simulink model "PrinterRC_SIM"  (Simulink 7.8)
settings: Solver=FixedStepDiscrete  StartTime=0.0  StopTime=30  FixedStep=1/1000  RelTol=1e-3
InitFcn:
  | load('Exp_RC_settings.mat');
values from neighbouring files (symbols this model uses):
  N = length(r)    [SimExpRC_SPERTE.m]
  N_RC_activate = 5    [SimExpRC_SPERTE.m]
  N_trial = 50    [SimExpRC_SPERTE.m]
  p_Q = M    (= 50)    [DesignControllerRC.m]
undefined symbols (not defined in the file or in its folder): p_L, r
libraries: simulink x4, cstblocks x3
settings Model: Creator=jbolder  LastModifiedBy=lblanken
settings DebuggingCC: FrameProcessingCompatibilityMsg=error
settings CodeAppCC: CustomSymbolStrType=$N$R$M_T
settings GRTTargetCC: TargetFunctionLibrary=C89/C90 (ANSI)

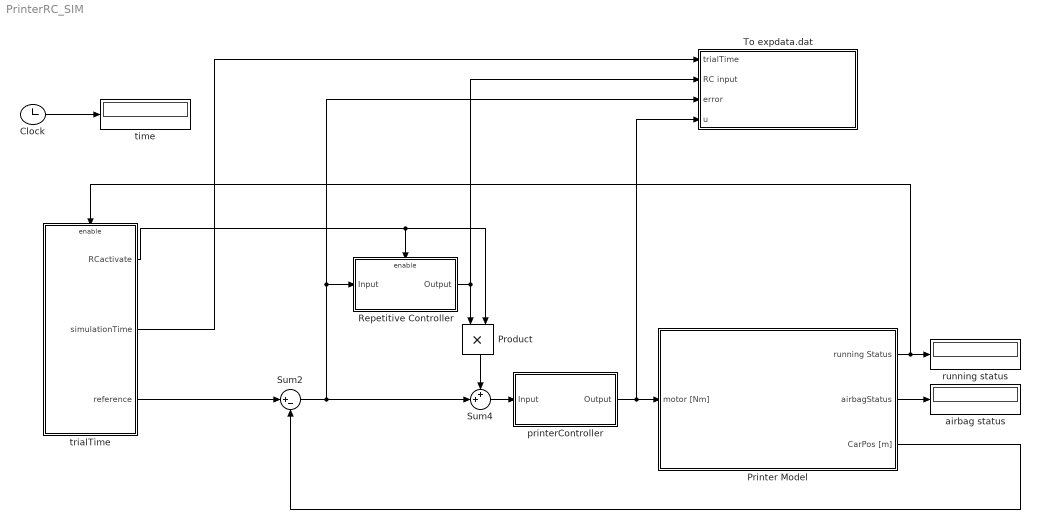
== system PrinterRC_SIM ==
  Clock : Clock
  Printer Model : Subsystem  InitFcn=load('PrinterModel.mat');
  Product : Product
  Repetitive Controller : Subsystem  InitFcn=load('RCController.mat');
  Sum2 : Sum  Inputs=|+-
  Sum4 : Sum  Inputs=++|  SaturateOnIntegerOverflow=on  InputSameDT=on  OutDataTypeStr=Inherit: Same as first input
  To expdata.dat : Subsystem
  airbag status : Display
      settings: Decimation=50
  printerController : Subsystem
  running status : Display
      settings: Decimation=50
  time : Display
      settings: Decimation=50
  trialTime : Subsystem  TreatAsAtomicUnit=on
  wires:
  trialTime/3(reference) -> Sum2/1
  Clock/1 -> time/1
  Printer Model/3(CarPos [m]) -> Sum2/2
  printerController/1(Output) -> To expdata.dat/4(u), Printer Model/1(motor [Nm])
  Printer Model/1(running Status) -> trialTime/Enable, running status/1
  Printer Model/2(airbagStatus) -> airbag status/1
  Sum4/1 -> printerController/1(Input)
  Repetitive Controller/1(Output) -> To expdata.dat/2(RC input), Product/1
  Sum2/1 -> Sum4/2, Repetitive Controller/1(Input), To expdata.dat/3(error)
  trialTime/2(simulationTime) -> To expdata.dat/1(trialTime)
  trialTime/1(RCactivate) -> Product/2, Repetitive Controller/Enable
  Product/1 -> Sum4/1

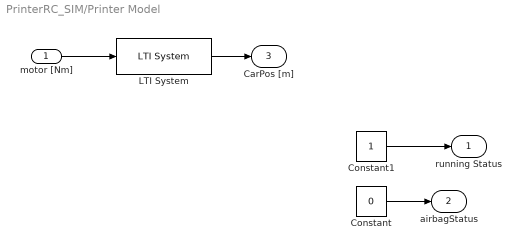
== system PrinterRC_SIM/Printer Model ==
  motor [Nm] : Inport
  Constant : Constant  Value=0
  Constant1 : Constant
  LTI System : cstblocks/LTI System  sys=PrinterModelSS  IC=[]
  running Status : Outport
  airbagStatus : Outport  Port=2
  CarPos [m] : Outport  Port=3
  wires:
  Constant1/1 -> running Status/1
  Constant/1 -> airbagStatus/1
  motor [Nm]/1 -> LTI System/1
  LTI System/1 -> CarPos [m]/1

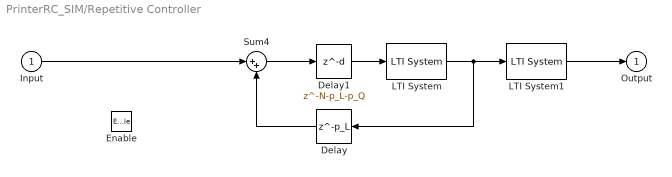
== system PrinterRC_SIM/Repetitive Controller ==
  Input : Inport
  Enable : EnablePort  StatesWhenEnabling=reset
  Delay : Delay  DelayLength=p_L  InitialCondition=0
  Delay1 : Delay  DelayLength=N-p_L-p_Q  InitialCondition=0
  LTI System : cstblocks/LTI System  sys=Q_c  IC=[]
  LTI System1 : cstblocks/LTI System  sys=L_c  IC=[]
  Sum4 : Sum  Inputs=|++  SaturateOnIntegerOverflow=on  InputSameDT=on  OutDataTypeStr=Inherit: Same as first input
  Output : Outport  InitialOutput=[0]
  wires:
  Input/1 -> Sum4/1
  LTI System1/1 -> Output/1
  Sum4/1 -> Delay1/1
  Delay/1 -> Sum4/2
  Delay1/1 -> LTI System/1
  LTI System/1 -> LTI System1/1, Delay/1

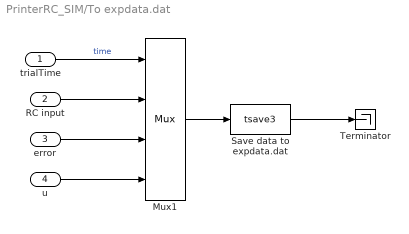
== system PrinterRC_SIM/To expdata.dat ==
  trialTime : Inport
  RC input : Inport  Port=2
  error : Inport  Port=3
  u : Inport  Port=4
  Mux1 : Mux
  Save data to expdata.dat : S-Function  FunctionName=tsave3  Parameters=0  SFunctionDeploymentMode=off  EnableBusSupport=off
  Terminator : Terminator
  wires:
  Mux1/1 -> Save data to expdata.dat/1
  Save data to expdata.dat/1 -> Terminator/1
  trialTime/1 -> Mux1/1  "time"
  RC input/1 -> Mux1/2
  error/1 -> Mux1/3
  u/1 -> Mux1/4

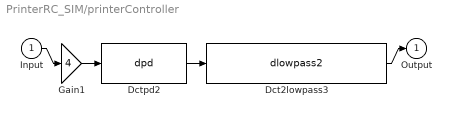
== system PrinterRC_SIM/printerController ==
  Input : Inport
  Dct2lowpass3 : S-Function  FunctionName=dlowpass2  Parameters=f_den, b_den, 0.001  SFunctionDeploymentMode=off  EnableBusSupport=off  mask(dctools){f_den=40, b_den=0.7}
      mask prompts: f_den "Pole [Hz]"; b_den "Damping pole [-]"
      mask help: This block implements a discrete time 2nd order lowpass filter.
      mask Display: disp('DCT 2nd order lowpass')
  Dctpd2 : S-Function  FunctionName=dpd  Parameters=kp, kv, 0.001  SFunctionDeploymentMode=off  EnableBusSupport=off  mask(dctools){kp=40, kv=1}
      mask help: This block implements a discrete time pd filter.
      mask Display: disp('DCT pd')
  Gain1 : Gain  Gain=4  SaturateOnIntegerOverflow=on  OutDataTypeStr=Inherit: Same as input  ParamDataTypeStr=Inherit: Same as input
  Output : Outport
  wires:
  Input/1 -> Gain1/1
  Gain1/1 -> Dctpd2/1
  Dctpd2/1 -> Dct2lowpass3/1
  Dct2lowpass3/1 -> Output/1

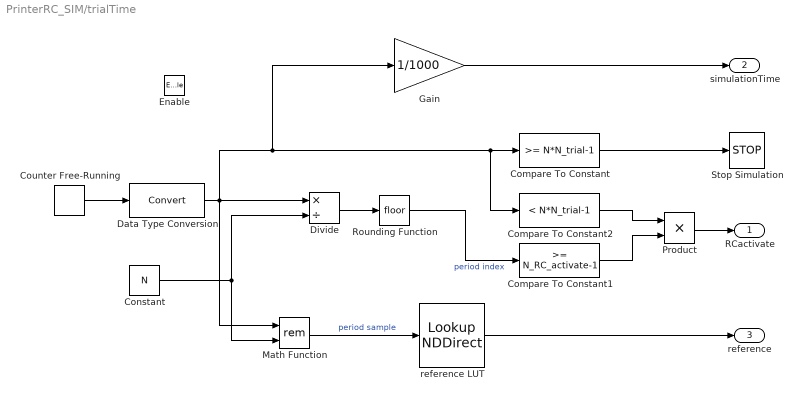
== system PrinterRC_SIM/trialTime ==
  Enable : EnablePort  StatesWhenEnabling=reset
  Compare To Constant : simulink/Logic and Bit Operations/Compare To Constant  relop=>=  const=N*N_trial-1  OutDataTypeStr=boolean
  Compare To Constant1 : simulink/Logic and Bit Operations/Compare To Constant  relop=>=  const=N_RC_activate-1  OutDataTypeStr=boolean
  Compare To Constant2 : simulink/Logic and Bit Operations/Compare To Constant  relop=<  const=N*N_trial-1  OutDataTypeStr=boolean
  Constant : Constant  Value=N
  Counter Free-Running : simulink/Sources/Counter Free-Running  NumBits=16  tsamp=-1
  Data Type Conversion : DataTypeConversion
  Divide : Product  Inputs=*/
  Gain : Gain  Gain=1/1000
  Math Function : Math  Operator=rem  SaturateOnIntegerOverflow=on
  Product : Product
  Rounding Function : Rounding
  Stop Simulation : Stop
  reference LUT : LookupNDDirect  NumberOfTableDimensions=1  Table=r
  RCactivate : Outport  InitialOutput=0
  simulationTime : Outport  Port=2  InitialOutput=0
  reference : Outport  Port=3  InitialOutput=0
  wires:
  Compare To Constant/1 -> Stop Simulation/1
  Math Function/1 -> reference LUT/1  "period sample"
  Counter Free-Running/1 -> Data Type Conversion/1
  Constant/1 -> Divide/2, Math Function/2
  Divide/1 -> Rounding Function/1
  Rounding Function/1 -> Compare To Constant1/1  "period index"
  Gain/1 -> simulationTime/1
  reference LUT/1 -> reference/1
  Compare To Constant1/1 -> Product/2
  Product/1 -> RCactivate/1
  Data Type Conversion/1 -> Divide/1, Gain/1, Compare To Constant2/1, Compare To Constant/1, Math Function/1
  Compare To Constant2/1 -> Product/1
